simulink library "INT_ErrLmp_VD"  (R2016b)
settings: Solver=VariableStepAuto  StartTime=0.0  StopTime=10.0  RelTol=1e-3
settings Model: Creator=lenovo  LastModifiedBy=lenovo

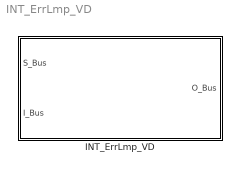
== system INT_ErrLmp_VD ==
  INT_ErrLmp_VD : Subsystem

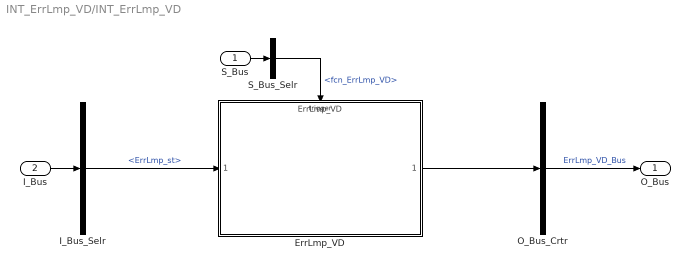
== system INT_ErrLmp_VD/INT_ErrLmp_VD ==
  S_Bus : Inport
  I_Bus : Inport  Port=2
  ErrLmp_VD : ModelReference  ModelNameDialog=ErrLmp_VD  SimulationMode=Normal  ModelReferenceVersion=1.3  TriggerPortName=function  TriggerPortTriggerType=function-call  TriggerPortStatesWhenEnabling=held
  I_Bus_Selr : BusSelector  OutputSignals=ErrLmp_st
  O_Bus_Crtr : BusCreator  Inputs=1
  S_Bus_Selr : BusSelector  OutputSignals=fcn_ErrLmp_VD
  O_Bus : Outport
  wires:
  S_Bus_Selr/1 -> ErrLmp_VD/Trigger  "<fcn_ErrLmp_VD>"
  S_Bus/1 -> S_Bus_Selr/1
  I_Bus/1 -> I_Bus_Selr/1
  I_Bus_Selr/1 -> ErrLmp_VD/1  "<ErrLmp_st>"
  O_Bus_Crtr/1 -> O_Bus/1  "ErrLmp_VD_Bus"
  ErrLmp_VD/1 -> O_Bus_Crtr/1
